simulink model "discrete_PID_pendulum"  (R2018a)
settings: Solver=ode5  StartTime=0.0  StopTime=50  FixedStep=0.01  MaxStep=0.01  RelTol=1e-3  EnableMultiTasking=on
values from neighbouring files (symbols this model uses):
  den = M_t*I_t - m^2*l^2*cos(theta_trim)    [PID_controller_design.m]    (also in unc_lin_model.m)
  f_c = ureal('f_c',0.5,'Percentage',20)    [PID_controller_design.m]    (also in unc_lin_model.m)
  f_p = ureal('f_p',6.65*10^(-5),'Percentage',20)    [PID_controller_design.m]    (also in unc_lin_model.m)
  g = 9.81    [PID_controller_design.m]    (also in unc_lin_model.m)
  I_t = I + m*l^2    [PID_controller_design.m]    (also in unc_lin_model.m)
  k_F = 12.86    [PID_controller_design.m]    (also in unc_lin_model.m)
  Ki_theta = par_pid(i,2)    [PID_robstab.m]    (also in PID_wcp.m; err_fun.m = par(:,2); sim_MC_PID.m = par_pid(3,2); sim_PID_pendulum_nominal.m = par_pid(3,2))
  Kp = par_pid(i,4)    [PID_robstab.m]    (also in PID_wcp.m; err_fun.m = par(:,4); sim_MC_PID.m = par_pid(3,4); sim_PID_pendulum_nominal.m = par_pid(3,4))
  Kp_theta = par_pid(i,1)    [PID_robstab.m]    (also in PID_wcp.m; err_fun.m = par(:,1); sim_MC_PID.m = par_pid(3,1); sim_PID_pendulum_nominal.m = par_pid(3,1))
  l = 0.174    [PID_controller_design.m]    (also in unc_lin_model.m)
  m = 0.104    [PID_controller_design.m]    (also in unc_lin_model.m)
  M_t = M + m    [PID_controller_design.m]    (also in unc_lin_model.m)
  N = par_pid(i,7)    [PID_robstab.m]    (also in PID_wcp.m; err_fun.m = par(:,7); sim_MC_PID.m = par_pid(3,7); sim_PID_pendulum_nominal.m = par_pid(3,7))
  N_theta = par_pid(i,6)    [PID_robstab.m]    (also in PID_wcp.m; err_fun.m = par(:,6); sim_MC_PID.m = par_pid(3,6); sim_PID_pendulum_nominal.m = par_pid(3,6))
  Td = par_pid(i,5)    [PID_robstab.m]    (also in PID_wcp.m; err_fun.m = par(:,5); sim_MC_PID.m = par_pid(3,5); sim_PID_pendulum_nominal.m = par_pid(3,5))
  Td_theta = par_pid(i,3)    [PID_robstab.m]    (also in PID_wcp.m; err_fun.m = par(:,3); sim_MC_PID.m = par_pid(3,3); sim_PID_pendulum_nominal.m = par_pid(3,3))
  u_max = 0.5    [PID_controller_design.m]    (also in PID_robstab.m; PID_wcp.m; sim_MC_PID.m; sim_PID_pendulum_nominal.m)
undefined symbols (not defined in the file or in its folder): DiscIntNeverNeededParam
libraries: simulink_extras x1
settings Model: Creator=ppetkov  LastModifiedBy=haykbeglaryan
settings DataIOCC: LimitDataPoints=on  SaveFormat=Array
settings OptimizationCC: ExpressionDepthLimit=2147483647  LifeSpan=inf
settings DebuggingCC: UnderspecifiedInitializationDetection=Classic  MergeDetectMultiDrivingBlocksExec=none  ParameterPrecisionLossMsg=none  FcnCallInpInsideContextMsg=warning  StateNameClashWarn=warning  SFUnexpectedBacktrackingDiag=warning  SFNoUnconditionalDefaultTransitionDiag=warning  SFExecutionAtInitializationDiag=none
settings HardwareCC: ProdBitPerPointer=32  ProdBitPerSizeT=32  ProdBitPerPtrDiffT=32  ProdLargestAtomicFloat=None  ProdIntDivRoundTo=Undefined  ProdEndianess=Unspecified  ProdWordSize=32  ProdHWDeviceType=32-bit Generic
settings ModelReferenceCC: PropagateSignalLabelsOutOfModel=off
settings CodeAppCC: StateflowObjectComments=on
settings GRTTargetCC: TargetLangStandard=C89/C90 (ANSI)  GeneratePreprocessorConditionals=Disable all  CombineOutputUpdateFcns=off  GRTInterface=on
settings ConfigComp: CovMetricSettings=dw  CovHtmlReporting=on  CovSaveCumulativeToWorkspaceVar=on  CovSaveSingleToWorkspaceVar=on  CovExternalEMLEnable=off

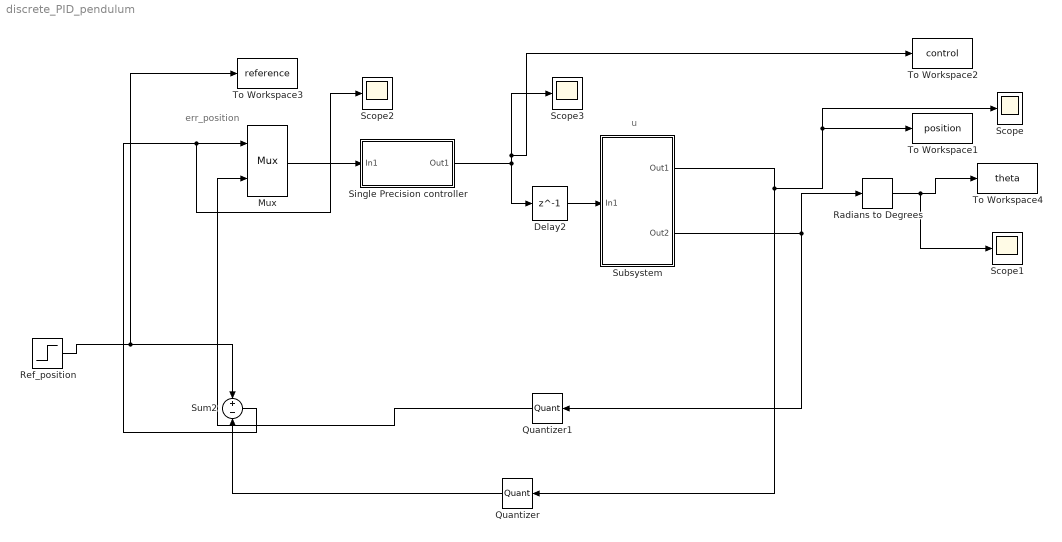
== system discrete_PID_pendulum ==
  note: err_position
  note: u
  Delay2 : Delay  DelayLength=1  SampleTime=0.01
  Mux : Mux  Inputs=2
  Quantizer : Quantizer  QuantizationInterval=0.235/2^12
  Quantizer1 : Quantizer  QuantizationInterval=2*pi/2^12
  Radians to Degrees : simulink_extras/Transformations/Radians to Degrees
  Ref_position : Step  Time=0  After=0.5  SampleTime=0
  Scope{,1..3} (4 alike) : Scope
  Single Precision controller : Subsystem
  Subsystem : Subsystem
  Sum2 : Sum  Inputs=+-
  To Workspace1 : ToWorkspace  VariableName=position  SampleTime=-1
      settings: Save2DSignal=2-D array (concatenate along first dimension)
  To Workspace2 : ToWorkspace  VariableName=control  SaveFormat=Structure With Time  SampleTime=-1
  To Workspace3 : ToWorkspace  VariableName=reference  SaveFormat=Structure With Time  SampleTime=-1
  To Workspace4 : ToWorkspace  VariableName=theta  SampleTime=-1
      settings: Save2DSignal=2-D array (concatenate along first dimension)
  wires:
  Mux/1 -> Single Precision controller/1(In1)
  Radians to Degrees/1 -> Scope1/1, To Workspace4/1
  Ref_position/1 -> Sum2/1, To Workspace3/1
  Sum2/1 -> Scope2/1, Mux/1
  Subsystem/1(Out1) -> To Workspace1/1, Scope/1, Quantizer/1
  Subsystem/2(Out2) -> Radians to Degrees/1, Quantizer1/1
  Single Precision controller/1(Out1) -> Delay2/1, To Workspace2/1, Scope3/1
  Delay2/1 -> Subsystem/1(In1)
  Quantizer/1 -> Sum2/2
  Quantizer1/1 -> Mux/2

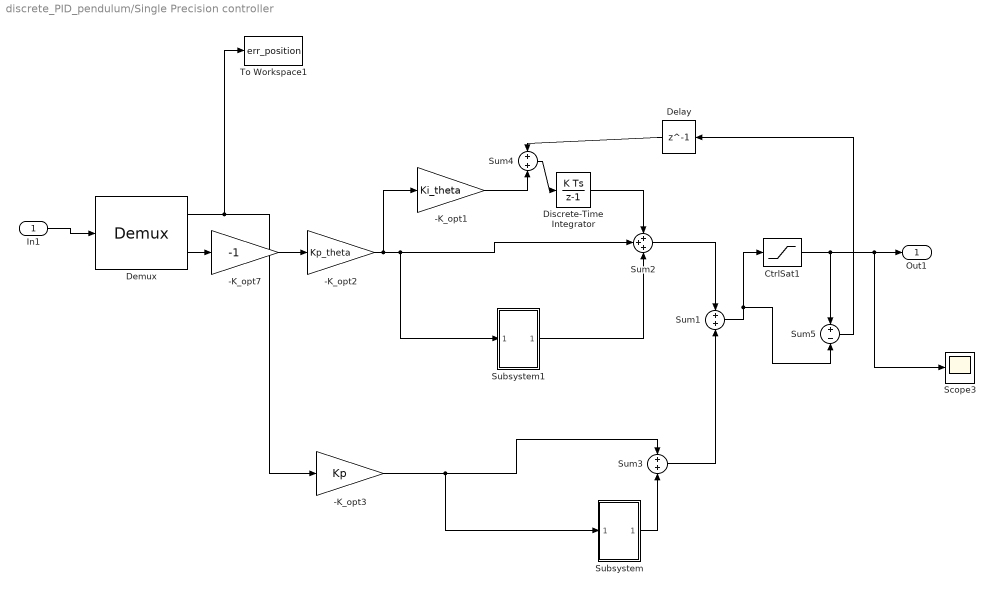
== system discrete_PID_pendulum/Single Precision controller ==
  In1 : Inport  OutDataTypeStr=double
  -K_opt1 : Gain  Gain=Ki_theta  OutDataTypeStr=double  RndMeth=Round  SaturateOnIntegerOverflow=on
  -K_opt2 : Gain  Gain=Kp_theta  OutDataTypeStr=double  RndMeth=Round  SaturateOnIntegerOverflow=on
  -K_opt3 : Gain  Gain=Kp  OutDataTypeStr=double  RndMeth=Round  SaturateOnIntegerOverflow=on
  -K_opt7 : Gain  Gain=-1  OutDataTypeStr=double  RndMeth=Round  SaturateOnIntegerOverflow=on
  CtrlSat1 : Saturate  UpperLimit=u_max  LowerLimit=-u_max  ZeroCross=off  OutDataTypeStr=double
  Delay : Delay  DelayLength=1  SampleTime=0.01
  Demux : Demux  Outputs=2
  Discrete-Time Integrator : DiscreteIntegrator  SampleTime=0.01  ICPrevOutput=DiscIntNeverNeededParam  ICPrevScaledInput=DiscIntNeverNeededParam
  Scope3 : Scope
  Subsystem : Subsystem
  Subsystem1 : Subsystem
  Sum1 : Sum
  Sum2 : Sum  Inputs=+++
  Sum3 : Sum
  Sum4 : Sum
  Sum5 : Sum  Inputs=+-
  To Workspace1 : ToWorkspace  VariableName=err_position  SampleTime=-1
      settings: Save2DSignal=2-D array (concatenate along first dimension)
  Out1 : Outport  OutDataTypeStr=double
  wires:
  Demux/1 -> To Workspace1/1, -K_opt3/1
  CtrlSat1/1 -> Scope3/1, Out1/1, Sum5/1
  In1/1 -> Demux/1
  Demux/2 -> -K_opt7/1
  Sum1/1 -> Sum5/2, CtrlSat1/1
  Sum2/1 -> Sum1/1
  -K_opt7/1 -> -K_opt2/1
  Discrete-Time Integrator/1 -> Sum2/1
  Subsystem1/1(Out1) -> Sum2/3
  -K_opt2/1 -> -K_opt1/1, Subsystem1/1(In1), Sum2/2
  Sum4/1 -> Discrete-Time Integrator/1
  -K_opt1/1 -> Sum4/2
  -K_opt3/1 -> Subsystem/1(In1), Sum3/1
  Subsystem/1(Out1) -> Sum3/2
  Sum3/1 -> Sum1/2
  Sum5/1 -> Delay/1
  Delay/1 -> Sum4/1

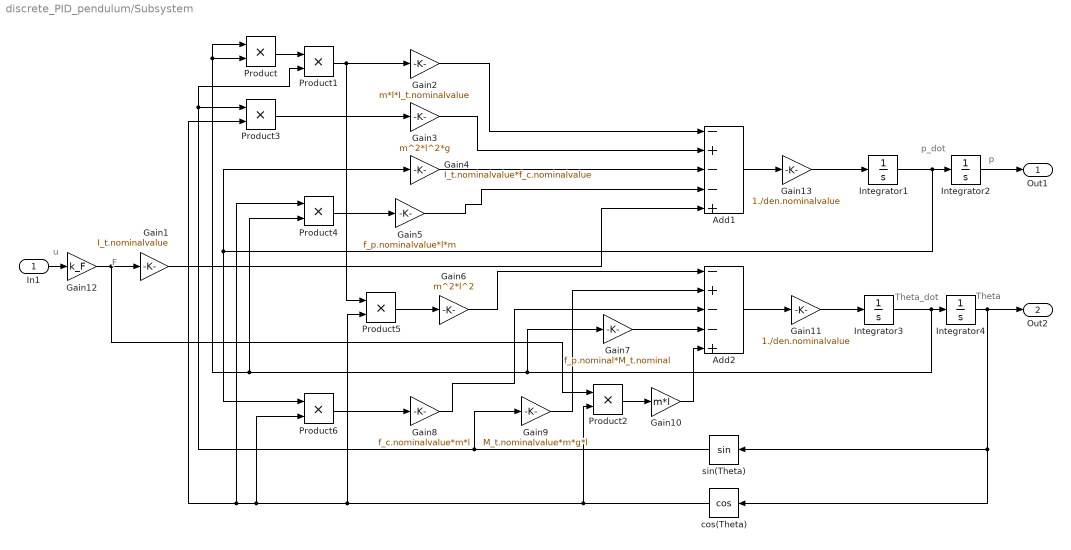
== system discrete_PID_pendulum/Subsystem ==
  note: p
  note: p_dot
  note: Theta
  note: Theta_dot
  note: F
  note: u
  In1 : Inport
  Add1 : Sum  Inputs=-+--+
  Add2 : Sum  Inputs=-+--+
  Gain1 : Gain  Gain=I_t.nominalvalue
  Gain10 : Gain  Gain=m*l
  Gain11 : Gain  Gain=1./den.nominalvalue
  Gain12 : Gain  Gain=k_F
  Gain13 : Gain  Gain=1./den.nominalvalue
  Gain2 : Gain  Gain=m*l*I_t.nominalvalue
  Gain3 : Gain  Gain=m^2*l^2*g
  Gain4 : Gain  Gain=I_t.nominalvalue*f_c.nominalvalue
  Gain5 : Gain  Gain=f_p.nominalvalue*l*m
  Gain6 : Gain  Gain=m^2*l^2
  Gain7 : Gain  Gain=f_p.nominal*M_t.nominal
  Gain8 : Gain  Gain=f_c.nominalvalue*m*l
  Gain9 : Gain  Gain=M_t.nominalvalue*m*g*l
  Integrator{1..4} (4 alike) : Integrator
  Product{,1..6} (7 alike) : Product  RndMeth=Zero
  cos(Theta) : Trigonometry  Operator=cos
  sin(Theta) : Trigonometry
  Out1 : Outport
  Out2 : Outport  Port=2
  wires:
  Integrator3/1 -> Integrator4/1, Gain7/1, Product4/2, Product/1, Product/2
  Product/1 -> Product1/1
  sin(Theta)/1 -> Gain9/1, Product3/1, Product1/2
  Add1/1 -> Gain13/1
  Gain13/1 -> Integrator1/1
  Gain4/1 -> Add1/3
  Product3/1 -> Gain3/1
  cos(Theta)/1 -> Product5/2, Product6/2, Product4/1, Product3/2, Product2/2
  Gain6/1 -> Add2/1
  Gain2/1 -> Add1/1
  Gain3/1 -> Add1/2
  Product5/1 -> Gain6/1
  Gain9/1 -> Add2/2
  Product1/1 -> Gain2/1, Product5/1
  Gain11/1 -> Integrator3/1
  Gain5/1 -> Add1/4
  Add2/1 -> Gain11/1
  Product4/1 -> Gain5/1
  Integrator2/1 -> Out1/1
  Integrator4/1 -> Out2/1, cos(Theta)/1, sin(Theta)/1
  Gain8/1 -> Add2/3
  Product6/1 -> Gain8/1
  Gain7/1 -> Add2/4
  Product2/1 -> Gain10/1
  Gain10/1 -> Add2/5
  Integrator1/1 -> Gain4/1, Product6/1, Integrator2/1
  Gain1/1 -> Add1/5
  In1/1 -> Gain12/1
  Gain12/1 -> Gain1/1, Product2/1

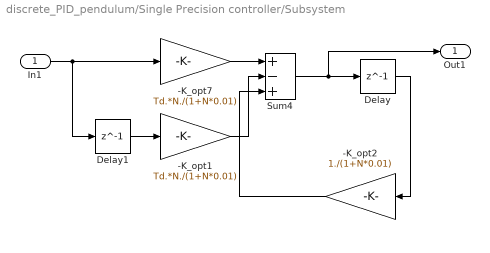
== system discrete_PID_pendulum/Single Precision controller/Subsystem ==
  In1 : Inport  OutDataTypeStr=double
  -K_opt1 : Gain  Gain=Td.*N./(1+N*0.01)  OutDataTypeStr=double  RndMeth=Round  SaturateOnIntegerOverflow=on
  -K_opt2 : Gain  Gain=1./(1+N*0.01)  OutDataTypeStr=double  RndMeth=Round  SaturateOnIntegerOverflow=on
  -K_opt7 : Gain  Gain=Td.*N./(1+N*0.01)  OutDataTypeStr=double  RndMeth=Round  SaturateOnIntegerOverflow=on
  Delay : Delay  DelayLength=1  SampleTime=0.01
  Delay1 : Delay  DelayLength=1  SampleTime=0.01
  Sum4 : Sum  Inputs=+-+
  Out1 : Outport  OutDataTypeStr=double
  wires:
  -K_opt2/1 -> Sum4/3
  Delay/1 -> -K_opt2/1
  -K_opt1/1 -> Sum4/2
  Sum4/1 -> Delay/1, Out1/1
  Delay1/1 -> -K_opt1/1
  -K_opt7/1 -> Sum4/1
  In1/1 -> -K_opt7/1, Delay1/1

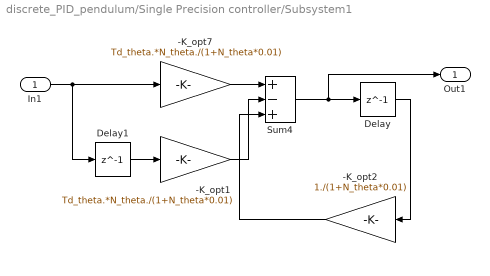
== system discrete_PID_pendulum/Single Precision controller/Subsystem1 ==
  In1 : Inport  OutDataTypeStr=double
  -K_opt1 : Gain  Gain=Td_theta.*N_theta./(1+N_theta*0.01)  OutDataTypeStr=double  RndMeth=Round  SaturateOnIntegerOverflow=on
  -K_opt2 : Gain  Gain=1./(1+N_theta*0.01)  OutDataTypeStr=double  RndMeth=Round  SaturateOnIntegerOverflow=on
  -K_opt7 : Gain  Gain=Td_theta.*N_theta./(1+N_theta*0.01)  OutDataTypeStr=double  RndMeth=Round  SaturateOnIntegerOverflow=on
  Delay : Delay  DelayLength=1  SampleTime=0.01
  Delay1 : Delay  DelayLength=1  SampleTime=0.01
  Sum4 : Sum  Inputs=+-+
  Out1 : Outport  OutDataTypeStr=double
  wires:
  In1/1 -> Delay1/1, -K_opt7/1
  -K_opt7/1 -> Sum4/1
  Delay1/1 -> -K_opt1/1
  Sum4/1 -> Out1/1, Delay/1
  -K_opt1/1 -> Sum4/2
  Delay/1 -> -K_opt2/1
  -K_opt2/1 -> Sum4/3
